simulink model "Project_P35_1"  (R2017b)
settings: Solver=VariableStepAuto  StartTime=0.0  StopTime=10.0  RelTol=1e-3
settings Model: Creator=Administrator  LastModifiedBy=Administrator

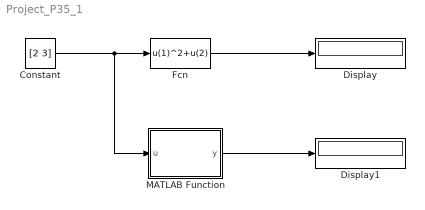
== system Project_P35_1 ==
  Constant : Constant  Value=[2 3]
  Display : Display
  Display1 : Display
  Fcn : Fcn  Expr=u(1)^2+u(2)
  MATLAB Function : MATLAB Function  TreatAsAtomicUnit=on
  wires:
  Fcn/1 -> Display/1
  MATLAB Function/1(y) -> Display1/1
  Constant/1 -> MATLAB Function/1(u), Fcn/1

== matlab function Project_P35_1/MATLAB Function ==
  data: u input; y output
function y = fcn(u)

y = max(u(1),u(2));
